simulink model "FABlock"  (R2025b)
settings: Solver=FixedStepDiscrete  StartTime=0.0  StopTime=4  RelTol=1e-3
settings Model: Creator=Soochan Kim  LastModifiedBy=Soochan Kim
settings OptimizationCC: BlockReduction=off  ConditionallyExecuteInputs=off  DefaultParameterBehavior=Inlined
settings DebuggingCC: SingleTaskRateTransMsg=error
settings HardwareCC: ProdBitPerPointer=32.0  ProdBitPerSizeT=32.0  ProdBitPerPtrDiffT=32.0  ProdLargestAtomicFloat=None  ProdIntDivRoundTo=Undefined  ProdEndianess=Unspecified  ProdWordSize=32.0  ProdHWDeviceType=ASIC/FPGA->ASIC/FPGA  TargetBitPerPointer=64.0  TargetBitPerSizeT=64.0  TargetBitPerPtrDiffT=64.0  TargetLongLongMode=on  TargetIntDivRoundTo=Zero  TargetEndianess=LittleEndian  TargetWordSize=64.0  TargetHWDeviceType=Custom Processor->MATLAB Host Computer  ProdEqTarget=off

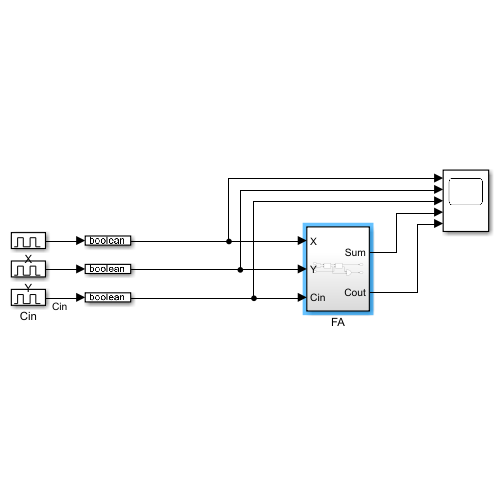
[thumbnail: Simulink's stored preview of the top-level diagram]
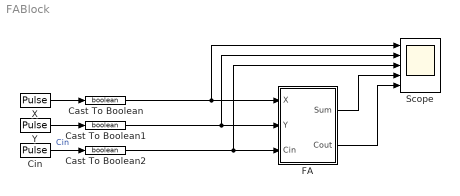
== system FABlock ==
  Cast To Boolean : DataTypeConversion  OutDataTypeStr=boolean  SaturateOnIntegerOverflow=off  RndMeth=Floor
  Cast To Boolean1 : DataTypeConversion  OutDataTypeStr=boolean  SaturateOnIntegerOverflow=off  RndMeth=Floor
  Cast To Boolean2 : DataTypeConversion  OutDataTypeStr=boolean  SaturateOnIntegerOverflow=off  RndMeth=Floor
  Cin : DiscretePulseGenerator  PulseType=Time based  Period=1  PulseWidth=50
  FA : Subsystem
  Scope : Scope  NumInputPorts=5
      settings: ActiveDisplayYMinimum=-0.12499999999999997  ActiveDisplayYMaximum=1.125
  X : DiscretePulseGenerator  PulseType=Time based  Period=1  PulseWidth=50
  Y : DiscretePulseGenerator  PulseType=Time based  Period=1  PulseWidth=50
  wires:
  Cin/1 -> Cast To Boolean2/1  "Cin"
  FA/1(Sum) -> Scope/4
  FA/2(Cout) -> Scope/5
  X/1 -> Cast To Boolean/1
  Y/1 -> Cast To Boolean1/1
  Cast To Boolean/1 -> Scope/1, FA/1(X)
  Cast To Boolean1/1 -> FA/2(Y), Scope/2
  Cast To Boolean2/1 -> Scope/3, FA/3(Cin)

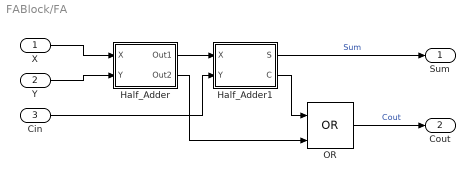
== system FABlock/FA ==
  X : Inport
  Y : Inport  Port=2
  Cin : Inport  Port=3
  Half_Adder : Subsystem  TreatAsAtomicUnit=on
  Half_Adder1 : Subsystem  TreatAsAtomicUnit=on
  OR : Logic  Operator=OR  IconShape=distinctive  AllPortsSameDT=off  OutDataTypeStr=boolean
  Sum : Outport
  Cout : Outport  Port=2
  wires:
  Half_Adder1/1(S) -> Sum/1  "Sum"
  OR/1 -> Cout/1  "Cout"
  X/1 -> Half_Adder/1(X)
  Y/1 -> Half_Adder/2(Y)
  Half_Adder/2(Out2) -> OR/2
  Cin/1 -> Half_Adder1/2(Y)
  Half_Adder/1(Out1) -> Half_Adder1/1(X)
  Half_Adder1/2(C) -> OR/1

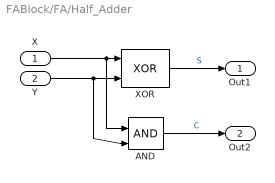
== system FABlock/FA/Half_Adder ==
  X : Inport
  Y : Inport  Port=2
  AND : Logic  IconShape=distinctive  AllPortsSameDT=off  OutDataTypeStr=boolean
  XOR : Logic  Operator=XOR  IconShape=distinctive  AllPortsSameDT=off  OutDataTypeStr=boolean
  Out1 : Outport
  Out2 : Outport  Port=2
  wires:
  Y/1 -> AND/2, XOR/2
  XOR/1 -> Out1/1  "S"
  AND/1 -> Out2/1  "C"
  X/1 -> AND/1, XOR/1

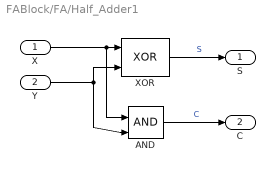
== system FABlock/FA/Half_Adder1 ==
  X : Inport
  Y : Inport  Port=2
  AND : Logic  IconShape=distinctive  AllPortsSameDT=off  OutDataTypeStr=boolean
  XOR : Logic  Operator=XOR  IconShape=distinctive  AllPortsSameDT=off  OutDataTypeStr=boolean
  S : Outport
  C : Outport  Port=2
  wires:
  Y/1 -> XOR/2, AND/2
  XOR/1 -> S/1  "S"
  AND/1 -> C/1  "C"
  X/1 -> AND/1, XOR/1
